simulink model "linax"  (R2019a)
settings: Solver=VariableStepAuto  StartTime=0.0  StopTime=1  RelTol=1e-3  EnableMultiTasking=on
model workspace (MATLAB code in the model file + MAT data in the model file):
  cmdLim = Simulink.Parameter
  cmdLim.Value = 15
  cmdLim.Description = 'Limit for controlling the maximum surface command angle.'
  cmdLim.Min = 0
  cmdLim.Max = 90
  cmdLim.DocUnits = 'deg'
  dispGain = Simulink.Parameter
  dispGain.Value = 0.75
  dispGain.Description = 'Gain applied to the displacement error.'
  dispGain.Min = 0
  dispGain.Max = []
  dispGain.DocUnits = 'deg/sec/deg'
  dispLim = Simulink.Parameter
  dispLim.Value = 30
  dispLim.Description = 'Limit for controlling the maximum commanded angle.'
  dispLim.Min = 0
  dispLim.Max = 180
  dispLim.DocUnits = 'deg'
  intGain = Simulink.Parameter
  intGain.Value = 0.5
  intGain.Description = 'Gain applied to the integral error.'
  intGain.Min = 0
  intGain.Max = []
  intGain.DocUnits = 'deg/sec/deg/sec'
  intLim = Simulink.Parameter
  intLim.Value = 5
  intLim.Description = 'Limit for controlling the maximum commanded angle.'
  intLim.Min = 0
  intLim.Max = 90
  intLim.DocUnits = 'deg'
  rateGain = Simulink.Parameter
  rateGain.Value = 2
  rateGain.Description = 'Gain applied to the rate error.'
  rateGain.Min = 0
  rateGain.Max = []
  rateGain.DocUnits = 'deg/deg/sec'
  rateLim = Simulink.Parameter
  rateLim.Value = 6
  rateLim.Description = 'Limit for controlling the maximum commanded angle.'
  rateLim.Min = 0
  rateLim.Max = 180
  rateLim.DocUnits = 'deg/sec'
  hdgGain = Simulink.Parameter
  hdgGain.Value = 0.015
  D = Simulink.Parameter
  D.Value = [5 5 5]
  D.Description = 'PID D'
  D.DataType = 'auto'
  D.Dimensions = [1 3]
  I = Simulink.Parameter
  I.Value = [11 11 11]
  I.Description = 'PID I'
  I.DataType = 'auto'
  I.Dimensions = [1 3]
  P = Simulink.Parameter
  P.Value = [2501 2001 2001]
  P.Description = 'PID P'
  P.DataType = 'auto'
  P.Dimensions = [1 3]
  c = Simulink.Parameter
  c.Value = [0.01 0.01 0.01]
  c.Description = 'Resistence'
  c.DataType = 'auto'
  c.Dimensions = [1 3]
  m = Simulink.Parameter
  m.Value = [1.5 1.1 1]
  m.Description = 'Mass'
  m.DataType = 'auto'
  m.Dimensions = [1 3]
  sat = Simulink.Parameter
  sat.Value = [3001 3000 3000]
  sat.Description = 'PID output saturation'
  sat.DataType = 'auto'
  sat.Dimensions = [1 3]
libraries: simulink x3
settings Model: RequirementInfo={} %GIDa_fe9045fd_0412_4b6e_8206_617cc20e6fde  FPTRunName=Active  OrderedModelArguments=off  Creator=p4010  LastModifiedBy=p4010
settings SolverCC: AutoInsertRateTranBlk=on
settings DataIOCC: SaveOutput=off  SignalLogging=off  DSMLogging=off  SaveTime=off
settings OptimizationCC: DefaultParameterBehavior=Inlined  UseDivisionForNetSlopeComputation=on  GainParamInheritBuiltInType=on  UseFloatMulNetSlope=on  UseSpecifiedMinMax=on  InlineInvariantSignals=on  PassReuseOutputArgsAs=Individual arguments  ZeroExternalMemoryAtStartup=off  ZeroInternalMemoryAtStartup=off  NoFixptDivByZeroProtection=on  EfficientFloat2IntCast=on  LifeSpan=1  OptimizeBlockOrder=speed  DifferentSizesBufferReuse=on
settings DebuggingCC: MultiTaskRateTransMsg=warning  AllowSymbolicDim=off  SFUnexpectedBacktrackingDiag=warning  SFNoUnconditionalDefaultTransitionDiag=warning  SFExecutionAtInitializationDiag=none  ArithmeticOperatorsInVariantConditions=warning
settings HardwareCC: ProdBitPerPointer=32  ProdBitPerSizeT=32  ProdBitPerPtrDiffT=32  ProdLargestAtomicInteger=Long  ProdWordSize=32  ProdLongLongMode=on  ProdHWDeviceType=ARM Compatible->ARM 7
settings SFSimCC: MATLABDynamicMemAlloc=off
settings RTWCC: SystemTargetFile=ert.tlc  GenCodeOnly=on  TemplateMakefile=ert_default_tmf  GenerateReport=on  BuildConfiguration=Faster Runs  IncludeHyperlinkInReport=on  LaunchReport=on  GenerateTraceInfo=on  GenerateTraceReport=on  GenerateTraceReportSl=on  GenerateTraceReportSf=on  GenerateTraceReportEml=on  GenerateCodeMetricsReport=on
settings CodeAppCC: ForceParamTrailComments=on  IgnoreCustomStorageClasses=off  OperatorAnnotations=on  SimulinkDataObjDesc=on  SFDataObjDesc=on  CustomSymbolStrGlobalVar=rt$N$M  CustomSymbolStrType=$N$M  CustomSymbolStrFcn=$N$M$F  CustomSymbolStrMacro=$N$M  InsertBlockDesc=on  EnableCustomComments=on  ReqsInCode=on
settings ERTTargetCC: TargetLangStandard=C99 (ISO)  UtilityFuncGeneration=Shared location  MultiwordLength=2048  GenerateSampleERTMain=on  IncludeMdlTerminateFcn=off  CombineSignalStateStructs=on  MultiInstanceERTCode=on  CodeInterfacePackaging=Reusable function  SupportNonFinite=off  SupportComplex=off  SupportContinuousTime=on  InlinedParameterPlacement=NonHierarchical  ERTCustomFileTemplate=example_file_process.tlc  ERTFilePackagingFormat=CompactWithDataFile
settings ConfigComp: CovScope=ReferencedModels  CovSaveName=covdata_rollAP  CovMetricSettings=dcmtrwe  CovHTMLOptions=-sRT=1 -aTS=1 -bRG=1 -bTC=1 -hTR=1 -nFC=0 -scm=1 -bcm=1 -xEv=0  CovSaveCumulativeToWorkspaceVar=on  CovSaveSingleToWorkspaceVar=on  CovCumulativeVarName=covCumulativeData_rollAP  CovReportOnPause=off  CovExternalEMLEnable=off  CovSFcnEnable=off

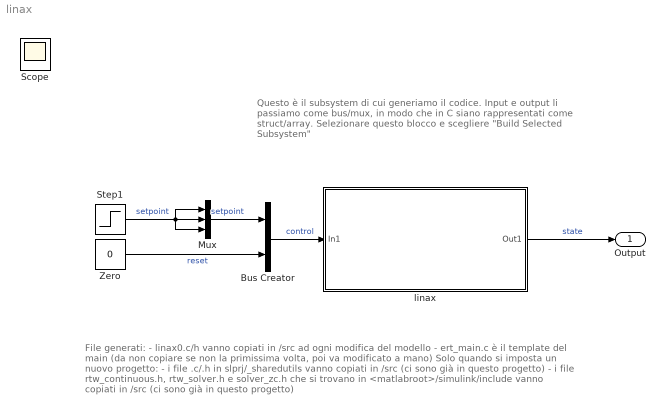
== system linax ==
  note: File generati:
      | - linax0.c/h vanno copiati in /src ad ogni modifica del modello
      | - ert_main.c è il template del main (da non copiare se non la primissima volta, poi va modificato a mano)
      | Solo quando si imposta un nuovo progetto:
      | - i file .c/.h in slprj/_sharedutils vanno copiati in /src (ci sono già in questo progetto)
      | - i file rtw_continuous.h, rtw_solver.h e solver_zc.h che si trovano in <matlabroot>/simulink/include vanno copiati in /src (ci sono già in questo progetto)
  note: Questo è il subsystem di cui generiamo il codice.
      | Input e output li passiamo come bus/mux,
      | in modo che in C siano rappresentati come struct/array.
      | Selezionare questo blocco e scegliere "Build Selected Subsystem"
  Bus Creator : BusCreator  Inputs=2
  Mux : Mux  Inputs=3
  Step1 : Step  Time=0.1  SampleTime=0.001
  Zero : Constant  Value=0  OutDataTypeStr=Inherit: Inherit via back propagation
  linax : Subsystem
  Output : Outport  SignalName=state
  Scope : Scope
  wires:
  Zero/1 -> Bus Creator/2  "reset"
  Bus Creator/1 -> linax/1(In1)  "control"
  linax/1(Out1) -> Output/1  "state"
  Mux/1 -> Bus Creator/1  "setpoint"
  Step1/1 -> Mux/3, Mux/2, Mux/1  "setpoint"

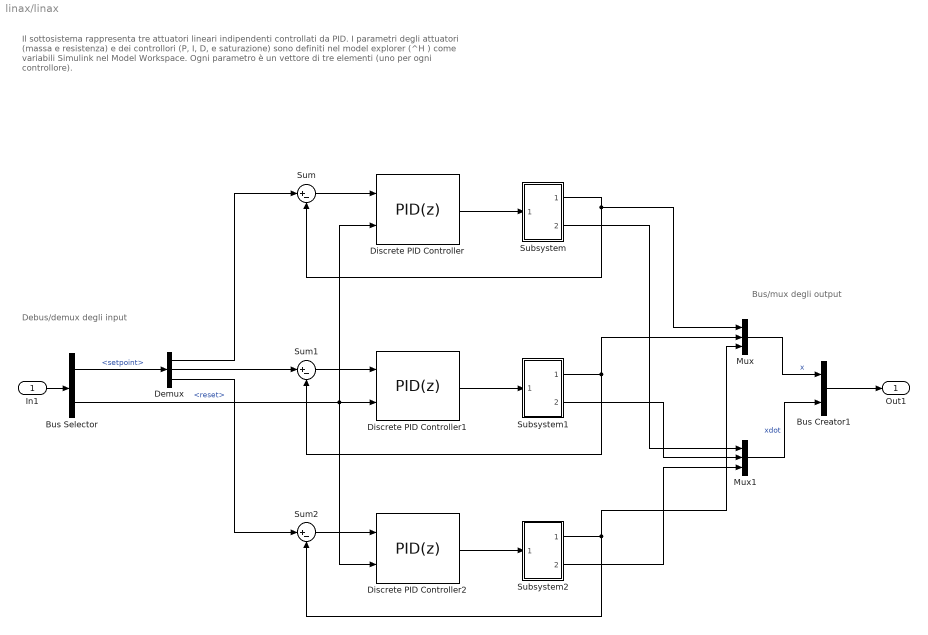
== system linax/linax ==
  note: Il sottosistema rappresenta tre attuatori lineari indipendenti controllati da PID.
      | I parametri degli attuatori (massa e resistenza) e dei controllori (P, I, D, e saturazione) sono definiti nel model explorer (^H )
      | come variabili Simulink nel Model Workspace.
      | Ogni parametro è un vettore di tre elementi (uno per ogni controllore).
  note: Bus/mux degli output
  note: Debus/demux degli input
  In1 : Inport
  Bus Creator1 : BusCreator  Inputs=2
  Bus Selector : BusSelector  OutputSignals=setpoint,reset
  Demux : Demux  Outputs=3
  Discrete PID Controller : simulink/Continuous/PID Controller  Controller=PID  Form=Parallel  TimeDomain=Discrete-time  SampleTime=0.005  IntegratorMethod=Forward Euler  FilterMethod=Forward Euler  ControllerParametersSource=internal  P=P(1)  I=I(1)  D=D(1)  UseFilter=off  N=163.464065982053  TunerSelectOption=Transfer Function Based (PID Tuner App)  InitialConditionSource=internal  InitialConditionForIntegrator=0  InitialConditionForFilter=0  DifferentiatorICPrevScaledInput=0  ExternalReset=rising  TrackingMode=off  Kt=1  LimitOutput=on  UpperSaturationLimit=sat(1)  LowerSaturationLimit=-sat(1)  LinearizeAsGain=off  AntiWindupMode=clamping  Kb=1  POutMin=[]  POutMax=[]  IOutMin=[]  IOutMax=[]  DOutMin=[]  DOutMax=[]  NOutMin=[]  NOutMax=[]  SumOutMin=[]  SumOutMax=[]  SaturationOutMin=[]  SaturationOutMax=[]  PParamMin=[]  PParamMax=[]  IParamMin=[]  IParamMax=[]  DParamMin=[]  DParamMax=[]  NParamMin=[]  NParamMax=[]  KbParamMin=[]  KbParamMax=[]  KtParamMin=[]  KtParamMax=[]  KbOutMin=[]  KbOutMax=[]  KtOutMin=[]  KtOutMax=[]  IntegratorOutMin=[]  IntegratorOutMax=[]  FilterOutMin=[]  FilterOutMax=[]  SumI1OutMin=[]  SumI1OutMax=[]  SumI2OutMin=[]  SumI2OutMax=[]  SumI3OutMin=[]  SumI3OutMax=[]  SumI4OutMin=[]  SumI4OutMax=[]  SumDOutMin=[]  SumDOutMax=[]  DifferentiatorOutMin=[]  DifferentiatorOutMax=[]  FilterDiffOutCoefMin=[]  FilterDiffOutCoefMax=[]  ReciprocalOutMin=[]  ReciprocalOutMax=[]  SumDenOutMin=[]  SumDenOutMax=[]  SumNumOutMin=[]  SumNumOutMax=[]  DivideOutMin=[]  DivideOutMax=[]  IntegratorContinuousStateAttributes=''  IntegratorStateMustResolveToSignalObject=off  IntegratorRTWStateStorageClass=Auto  FilterContinuousStateAttributes=''  FilterStateMustResolveToSignalObject=off  FilterRTWStateStorageClass=Auto  ParallelPVariant=InternalParameters  IdealPVariant=Disabled  IVariant=InternalParameters  DVariant=InternalParameters  IntegratorVariant=Discrete  SatVariant=Enabled  AWVariant=DiscClampingParallel  PCopyVariant=Disabled  TRVariant=Disabled  FdbkBlocksVariant=Forward  IdealPFdbkVariant=Disabled  SatFdbkVariant=Disabled  DerivativeFilterVariant=Differentiator  NVariant=Passthrough  NCopyVariant=Disabled_SignalSpec  FilterICVariant=InternalICsDifferentiator  IntegratorICVariant=InternalICs  ExternalResetVariant=ExternalReset  TRSumVariant=Passthrough  SumFdbkVariant=Disabled  SumVariant=Sum_PID
  Discrete PID Controller1 : simulink/Continuous/PID Controller  Controller=PID  Form=Parallel  TimeDomain=Discrete-time  SampleTime=0.005  IntegratorMethod=Forward Euler  FilterMethod=Forward Euler  ControllerParametersSource=internal  P=P(2)  I=I(2)  D=D(2)  UseFilter=off  N=163.464065982053  TunerSelectOption=Transfer Function Based (PID Tuner App)  InitialConditionSource=internal  InitialConditionForIntegrator=0  InitialConditionForFilter=0  DifferentiatorICPrevScaledInput=0  ExternalReset=rising  TrackingMode=off  Kt=1  LimitOutput=on  UpperSaturationLimit=sat(2)  LowerSaturationLimit=-sat(2)  LinearizeAsGain=off  AntiWindupMode=clamping  Kb=1  POutMin=[]  POutMax=[]  IOutMin=[]  IOutMax=[]  DOutMin=[]  DOutMax=[]  NOutMin=[]  NOutMax=[]  SumOutMin=[]  SumOutMax=[]  SaturationOutMin=[]  SaturationOutMax=[]  PParamMin=[]  PParamMax=[]  IParamMin=[]  IParamMax=[]  DParamMin=[]  DParamMax=[]  NParamMin=[]  NParamMax=[]  KbParamMin=[]  KbParamMax=[]  KtParamMin=[]  KtParamMax=[]  KbOutMin=[]  KbOutMax=[]  KtOutMin=[]  KtOutMax=[]  IntegratorOutMin=[]  IntegratorOutMax=[]  FilterOutMin=[]  FilterOutMax=[]  SumI1OutMin=[]  SumI1OutMax=[]  SumI2OutMin=[]  SumI2OutMax=[]  SumI3OutMin=[]  SumI3OutMax=[]  SumI4OutMin=[]  SumI4OutMax=[]  SumDOutMin=[]  SumDOutMax=[]  DifferentiatorOutMin=[]  DifferentiatorOutMax=[]  FilterDiffOutCoefMin=[]  FilterDiffOutCoefMax=[]  ReciprocalOutMin=[]  ReciprocalOutMax=[]  SumDenOutMin=[]  SumDenOutMax=[]  SumNumOutMin=[]  SumNumOutMax=[]  DivideOutMin=[]  DivideOutMax=[]  IntegratorContinuousStateAttributes=''  IntegratorStateMustResolveToSignalObject=off  IntegratorRTWStateStorageClass=Auto  FilterContinuousStateAttributes=''  FilterStateMustResolveToSignalObject=off  FilterRTWStateStorageClass=Auto  ParallelPVariant=InternalParameters  IdealPVariant=Disabled  IVariant=InternalParameters  DVariant=InternalParameters  IntegratorVariant=Discrete  SatVariant=Enabled  AWVariant=DiscClampingParallel  PCopyVariant=Disabled  TRVariant=Disabled  FdbkBlocksVariant=Forward  IdealPFdbkVariant=Disabled  SatFdbkVariant=Disabled  DerivativeFilterVariant=Differentiator  NVariant=Passthrough  NCopyVariant=Disabled_SignalSpec  FilterICVariant=InternalICsDifferentiator  IntegratorICVariant=InternalICs  ExternalResetVariant=ExternalReset  TRSumVariant=Passthrough  SumFdbkVariant=Disabled  SumVariant=Sum_PID
  Discrete PID Controller2 : simulink/Continuous/PID Controller  Controller=PID  Form=Parallel  TimeDomain=Discrete-time  SampleTime=0.005  IntegratorMethod=Forward Euler  FilterMethod=Forward Euler  ControllerParametersSource=internal  P=P(3)  I=I(3)  D=D(3)  UseFilter=off  N=163.464065982053  TunerSelectOption=Transfer Function Based (PID Tuner App)  InitialConditionSource=internal  InitialConditionForIntegrator=0  InitialConditionForFilter=0  DifferentiatorICPrevScaledInput=0  ExternalReset=rising  TrackingMode=off  Kt=1  LimitOutput=on  UpperSaturationLimit=sat(3)  LowerSaturationLimit=-sat(3)  LinearizeAsGain=off  AntiWindupMode=clamping  Kb=1  POutMin=[]  POutMax=[]  IOutMin=[]  IOutMax=[]  DOutMin=[]  DOutMax=[]  NOutMin=[]  NOutMax=[]  SumOutMin=[]  SumOutMax=[]  SaturationOutMin=[]  SaturationOutMax=[]  PParamMin=[]  PParamMax=[]  IParamMin=[]  IParamMax=[]  DParamMin=[]  DParamMax=[]  NParamMin=[]  NParamMax=[]  KbParamMin=[]  KbParamMax=[]  KtParamMin=[]  KtParamMax=[]  KbOutMin=[]  KbOutMax=[]  KtOutMin=[]  KtOutMax=[]  IntegratorOutMin=[]  IntegratorOutMax=[]  FilterOutMin=[]  FilterOutMax=[]  SumI1OutMin=[]  SumI1OutMax=[]  SumI2OutMin=[]  SumI2OutMax=[]  SumI3OutMin=[]  SumI3OutMax=[]  SumI4OutMin=[]  SumI4OutMax=[]  SumDOutMin=[]  SumDOutMax=[]  DifferentiatorOutMin=[]  DifferentiatorOutMax=[]  FilterDiffOutCoefMin=[]  FilterDiffOutCoefMax=[]  ReciprocalOutMin=[]  ReciprocalOutMax=[]  SumDenOutMin=[]  SumDenOutMax=[]  SumNumOutMin=[]  SumNumOutMax=[]  DivideOutMin=[]  DivideOutMax=[]  IntegratorContinuousStateAttributes=''  IntegratorStateMustResolveToSignalObject=off  IntegratorRTWStateStorageClass=Auto  FilterContinuousStateAttributes=''  FilterStateMustResolveToSignalObject=off  FilterRTWStateStorageClass=Auto  ParallelPVariant=InternalParameters  IdealPVariant=Disabled  IVariant=InternalParameters  DVariant=InternalParameters  IntegratorVariant=Discrete  SatVariant=Enabled  AWVariant=DiscClampingParallel  PCopyVariant=Disabled  TRVariant=Disabled  FdbkBlocksVariant=Forward  IdealPFdbkVariant=Disabled  SatFdbkVariant=Disabled  DerivativeFilterVariant=Differentiator  NVariant=Passthrough  NCopyVariant=Disabled_SignalSpec  FilterICVariant=InternalICsDifferentiator  IntegratorICVariant=InternalICs  ExternalResetVariant=ExternalReset  TRSumVariant=Passthrough  SumFdbkVariant=Disabled  SumVariant=Sum_PID
  Mux : Mux  Inputs=3
  Mux1 : Mux  Inputs=3
  Subsystem : Subsystem  mask{mass=m(1), resist=c(1)}
      mask prompts: resist "Resistence"
  Subsystem1 : Subsystem  mask{mass=m(2), resist=c(2)}
      mask prompts: resist "Resistence"
  Subsystem2 : Subsystem  mask{mass=m(3), resist=c(3)}
      mask prompts: resist "Resistence"
  Sum : Sum  Inputs=|+-
  Sum1 : Sum  Inputs=|+-
  Sum2 : Sum  Inputs=|+-
  Out1 : Outport
  wires:
  Subsystem/2(Output1) -> Mux1/1
  Bus Selector/2 -> Discrete PID Controller/2, Discrete PID Controller1/2, Discrete PID Controller2/2  "<reset>"
  In1/1 -> Bus Selector/1
  Bus Creator1/1 -> Out1/1
  Discrete PID Controller/1 -> Subsystem/1(In1)
  Subsystem/1(Output) -> Sum/2, Mux/1
  Sum/1 -> Discrete PID Controller/1
  Subsystem1/2(Output1) -> Mux1/2
  Discrete PID Controller1/1 -> Subsystem1/1(In1)
  Subsystem1/1(Output) -> Mux/2, Sum1/2
  Sum1/1 -> Discrete PID Controller1/1
  Subsystem2/2(Output1) -> Mux1/3
  Discrete PID Controller2/1 -> Subsystem2/1(In1)
  Subsystem2/1(Output) -> Mux/3, Sum2/2
  Sum2/1 -> Discrete PID Controller2/1
  Bus Selector/1 -> Demux/1  "<setpoint>"
  Demux/1 -> Sum/1
  Demux/2 -> Sum1/1
  Demux/3 -> Sum2/1
  Mux/1 -> Bus Creator1/1  "x"
  Mux1/1 -> Bus Creator1/2  "xdot"

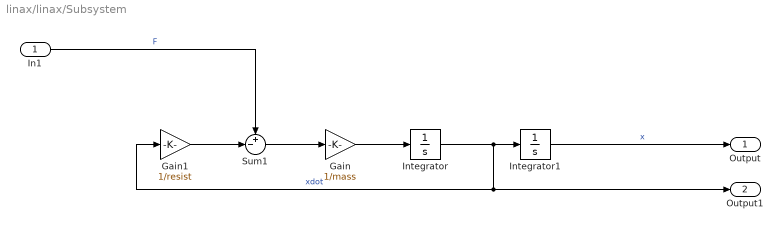
== system linax/linax/Subsystem ==
  In1 : Inport
  Gain : Gain  Gain=1/mass
  Gain1 : Gain  Gain=1/resist
  Integrator : Integrator
  Integrator1 : Integrator
  Sum1 : Sum  Inputs=+-|
  Output : Outport
  Output1 : Outport  Port=2
  wires:
  In1/1 -> Sum1/1  "F"
  Integrator1/1 -> Output/1  "x"
  Gain1/1 -> Sum1/2
  Sum1/1 -> Gain/1
  Integrator/1 -> Output1/1, Gain1/1, Integrator1/1  "xdot"
  Gain/1 -> Integrator/1

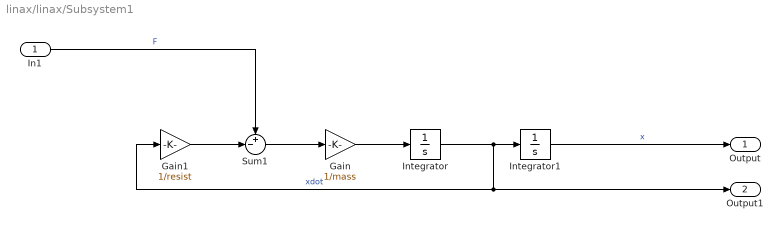
== system linax/linax/Subsystem1 ==
  In1 : Inport
  Gain : Gain  Gain=1/mass
  Gain1 : Gain  Gain=1/resist
  Integrator : Integrator
  Integrator1 : Integrator
  Sum1 : Sum  Inputs=+-|
  Output : Outport
  Output1 : Outport  Port=2
  wires:
  In1/1 -> Sum1/1  "F"
  Integrator1/1 -> Output/1  "x"
  Gain1/1 -> Sum1/2
  Sum1/1 -> Gain/1
  Integrator/1 -> Output1/1, Gain1/1, Integrator1/1  "xdot"
  Gain/1 -> Integrator/1

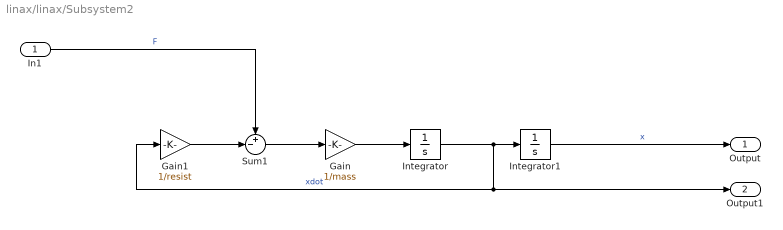
== system linax/linax/Subsystem2 ==
  In1 : Inport
  Gain : Gain  Gain=1/mass
  Gain1 : Gain  Gain=1/resist
  Integrator : Integrator
  Integrator1 : Integrator
  Sum1 : Sum  Inputs=+-|
  Output : Outport
  Output1 : Outport  Port=2
  wires:
  In1/1 -> Sum1/1  "F"
  Integrator1/1 -> Output/1  "x"
  Gain1/1 -> Sum1/2
  Sum1/1 -> Gain/1
  Integrator/1 -> Output1/1, Gain1/1, Integrator1/1  "xdot"
  Gain/1 -> Integrator/1
